simulink model "zadanie3"  (R2020a)
settings: Solver=FixedStepAuto  StartTime=0.0  StopTime=40  FixedStep=0.005  RelTol=1e-3
values from neighbouring files (symbols this model uses):
  ki = k_i(j)    [zadanie3_skrypt.m]
  kp_2 = 3    [zadanie3_skrypt.m]
undefined symbols (not defined in the file or in its folder): kp
settings Model: Creator=L1.3-21_2  LastModifiedBy=admin
settings DataIOCC: ReturnWorkspaceOutputs=off
settings DebuggingCC: ArithmeticOperatorsInVariantConditions=warning
settings SFSimCC: SimUseLocalCustomCode=off  CustomCodeUndefinedFunction=UseInterfaceOnly
settings RTWCC: RTWUseLocalCustomCode=off

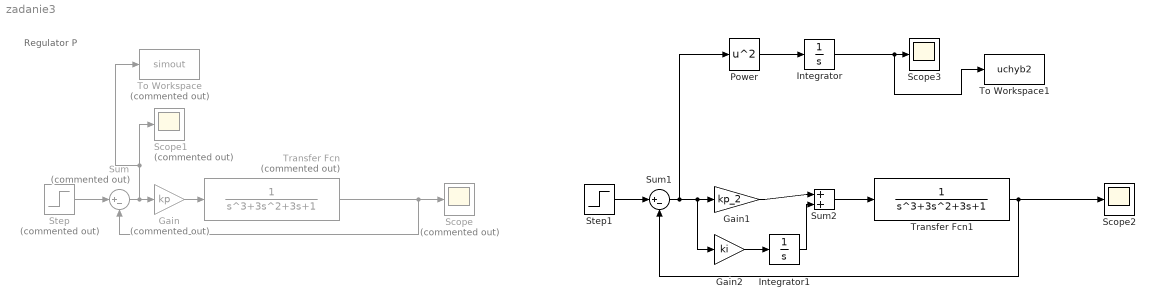
== system zadanie3 ==
  note: Regulator P
  Gain : Gain  Commented=on  Gain=kp
  Gain1 : Gain  Gain=kp_2
  Gain2 : Gain  Gain=ki
  Integrator : Integrator
  Integrator1 : Integrator
  Power : Math  Operator=square  SaturateOnIntegerOverflow=on
  Scope : Scope  Commented=on
  Scope1 : Scope  Commented=on
  Scope2 : Scope
  Scope3 : Scope
  Step : Step  Commented=on  SampleTime=0
  Step1 : Step  SampleTime=0
  Sum : Sum  Commented=on  Inputs=|+-
  Sum1 : Sum  Inputs=|+-
  Sum2 : Sum  Inputs=|++
  To Workspace : ToWorkspace  Commented=on  VariableName=simout  SaveFormat=Timeseries  SampleTime=-1
  To Workspace1 : ToWorkspace  VariableName=uchyb2  SaveFormat=Timeseries  SampleTime=-1
  Transfer Fcn : TransferFcn  Commented=on  Denominator=[1 3 3 1]
  Transfer Fcn1 : TransferFcn  Denominator=[1 3 3 1]
  wires:
  Transfer Fcn/1 -> Sum/2, Scope/1
  Gain/1 -> Transfer Fcn/1
  Sum/1 -> To Workspace/1, Scope1/1, Gain/1
  Step/1 -> Sum/1
  Step1/1 -> Sum1/1
  Transfer Fcn1/1 -> Sum1/2, Scope2/1
  Sum1/1 -> Power/1, Gain2/1, Gain1/1
  Power/1 -> Integrator/1
  Integrator/1 -> To Workspace1/1, Scope3/1
  Gain2/1 -> Integrator1/1
  Gain1/1 -> Sum2/1
  Integrator1/1 -> Sum2/2
  Sum2/1 -> Transfer Fcn1/1
